simulink model "autopilot"  (R2022b)
settings: Solver=VariableStepAuto  StartTime=0.0  StopTime=1000  RelTol=1e-3
libraries: mssSimulink x1
settings Model: Creator=XinyiWu  LastModifiedBy=ADMIN
settings ModelReferenceCC: EnableRefExpFcnMdlSchedulingChecks=on

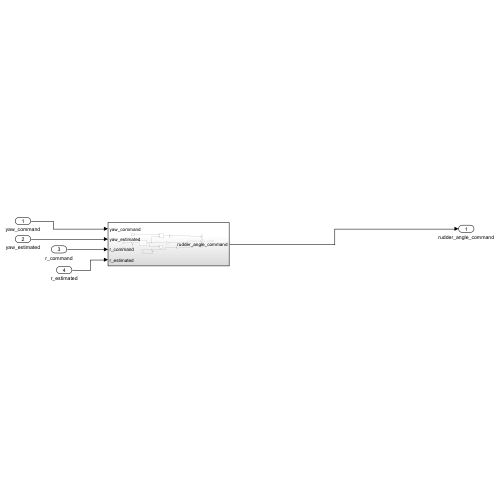
[thumbnail: Simulink's stored preview of the top-level diagram]
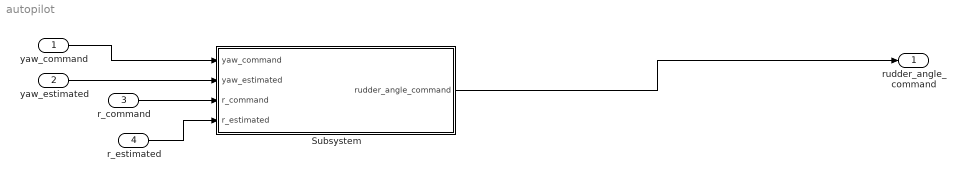
== system autopilot ==
  yaw_command : Inport
  yaw_estimated : Inport  Port=2
  r_command : Inport  Port=3
  r_estimated : Inport  Port=4
  Subsystem : Subsystem
  rudder_angle_command : Outport
  wires:
  yaw_command/1 -> Subsystem/1(yaw_command)
  yaw_estimated/1 -> Subsystem/2(yaw_estimated)
  r_command/1 -> Subsystem/3(r_command)
  r_estimated/1 -> Subsystem/4(r_estimated)
  Subsystem/1(rudder_angle_command) -> rudder_angle_command/1

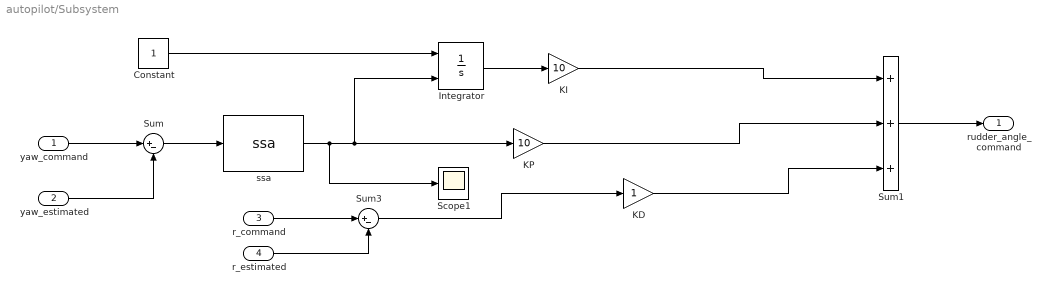
== system autopilot/Subsystem ==
  yaw_command : Inport
  yaw_estimated : Inport  Port=2
  r_command : Inport  Port=3
  r_estimated : Inport  Port=4
  Constant : Constant
  Integrator : Integrator  ExternalReset=level hold  LimitOutput=on  UpperSaturationLimit=20  LowerSaturationLimit=-20
  KD : Gain
  KI : Gain  Gain=10
  KP : Gain  Gain=10
  Scope1 : Scope
  Sum : Sum  Inputs=|+-
  Sum1 : Sum  Inputs=+++  InputSameDT=on  SaturateOnIntegerOverflow=on  OutDataTypeStr=Inherit: Same as first input
  Sum3 : Sum  Inputs=|+-  InputSameDT=on  SaturateOnIntegerOverflow=on  OutDataTypeStr=Inherit: Same as first input
  "ssa " : mssSimulink/Utilities/Math Operations/ssa  SystemSampleTime=-1  VariantActivationTime=update diagram  Latency=0  AutoFrameSizeCalculation=off
  rudder_angle_command : Outport
  wires:
  Integrator/1 -> KI/1
  KD/1 -> Sum1/3
  Constant/1 -> Integrator/1
  KP/1 -> Sum1/2
  Sum/1 -> "ssa "/1
  Sum3/1 -> KD/1
  "ssa "/1 -> Scope1/1, Integrator/2, KP/1
  KI/1 -> Sum1/1
  Sum1/1 -> rudder_angle_command/1
  r_estimated/1 -> Sum3/2
  r_command/1 -> Sum3/1
  yaw_command/1 -> Sum/1
  yaw_estimated/1 -> Sum/2
